simulink model "drone_sim"  (R2022a)
settings: Solver=VariableStepAuto  StartTime=0.0  StopTime=100  RelTol=1e-3
libraries: slpidlib x3
settings Model: Creator=jovanny-macbookair  LastModifiedBy=jovanny-macbookair

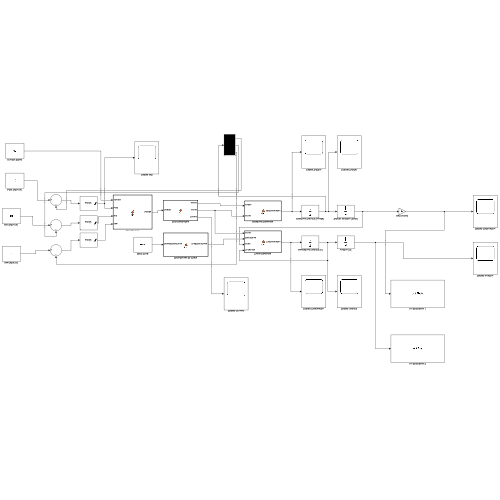
[thumbnail: Simulink's stored preview of the top-level diagram]
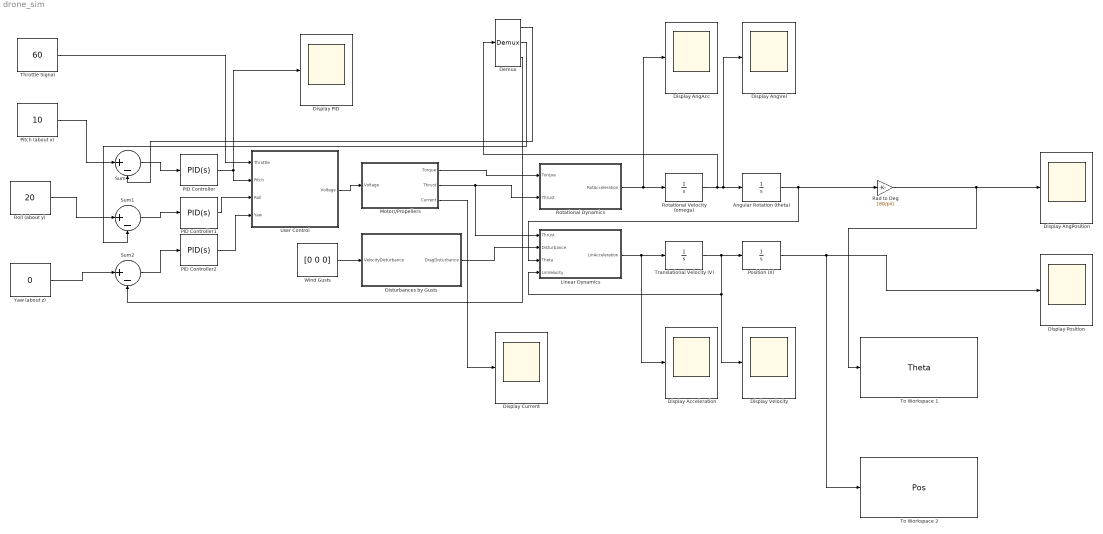
== system drone_sim ==
  Angular Rotation (theta) : Integrator
  Demux : Demux  Outputs=3
  Display Acceleration : Scope
  Display AngAcc : Scope
  Display AngPosition : Scope
  Display AngVel : Scope
  Display Current : Scope
  Display PID : Scope
  Display Position : Scope
  Display Velocity : Scope
  Disturbances by Gusts : MATLAB Function  TreatAsAtomicUnit=on
  Linear Dynamics : MATLAB Function  TreatAsAtomicUnit=on
  Motor//Propellers : MATLAB Function  TreatAsAtomicUnit=on
  PID Controller : slpidlib/PID Controller  Controller=PID  Form=Parallel  TimeDomain=Continuous-time  UseExternalTs=off  SampleTime=-1  IntegratorMethod=Forward Euler  FilterMethod=Forward Euler  ControllerParametersSource=internal  P=10  I=5  UseKiTs=off  D=0  N=100  UseFilter=on  TunerSelectOption=Transfer Function Based (PID Tuner App)  InitialConditionSource=internal  InitialConditionForIntegrator=0  InitialConditionForFilter=0  DifferentiatorICPrevScaledInput=0  ExternalReset=none  TrackingMode=off  Kt=1  LimitOutput=on  SatLimitsSource=internal  UpperSaturationLimit=100  LowerSaturationLimit=0  LinearizeAsGain=on  AntiWindupMode=clamping  Kb=1  POutMin=[]  POutMax=[]  IOutMin=[]  IOutMax=[]  DOutMin=[]  DOutMax=[]  NOutMin=[]  NOutMax=[]  SumOutMin=[]  SumOutMax=[]  SaturationOutMin=[]  SaturationOutMax=[]  PParamMin=[]  PParamMax=[]  IParamMin=[]  IParamMax=[]  DParamMin=[]  DParamMax=[]  NParamMin=[]  NParamMax=[]  KbParamMin=[]  KbParamMax=[]  KtParamMin=[]  KtParamMax=[]  KbOutMin=[]  KbOutMax=[]  KtOutMin=[]  KtOutMax=[]  IntegratorOutMin=[]  IntegratorOutMax=[]  FilterOutMin=[]  FilterOutMax=[]  SumI1OutMin=[]  SumI1OutMax=[]  SumI2OutMin=[]  SumI2OutMax=[]  SumI3OutMin=[]  SumI3OutMax=[]  SumI4OutMin=[]  SumI4OutMax=[]  SumDOutMin=[]  SumDOutMax=[]  DifferentiatorOutMin=[]  DifferentiatorOutMax=[]  FilterDiffOutCoefMin=[]  FilterDiffOutCoefMax=[]  ReciprocalOutMin=[]  ReciprocalOutMax=[]  SumDenOutMin=[]  SumDenOutMax=[]  SumNumOutMin=[]  SumNumOutMax=[]  DivideOutMin=[]  DivideOutMax=[]  UdiffTsProdOutMin=[]  UdiffTsProdOutMax=[]  NTsProdOutMin=[]  NTsProdOutMax=[]  UintegralTsProdOutMin=[]  UintegralTsProdOutMax=[]  UngainTsProdOutMin=[]  UngainTsProdOutMax=[]  IntegratorContinuousStateAttributes=''  IntegratorStateMustResolveToSignalObject=off  IntegratorRTWStateStorageClass=Auto  FilterContinuousStateAttributes=''  FilterStateMustResolveToSignalObject=off  FilterRTWStateStorageClass=Auto  ParallelPVariant=InternalParameters  IdealPVariant=Disabled  IVariant=InternalParameters  DVariant=InternalParameters  IntegratorVariant=Continuous  SatVariant=Enabled  AWVariant=ContClampingParallel  PCopyVariant=Disabled  TRVariant=Disabled  FdbkBlocksVariant=Forward  IdealPFdbkVariant=Disabled  SatFdbkVariant=Disabled  DerivativeFilterVariant=ContFilter  NVariant=InternalParameters  NCopyVariant=Disabled  FilterICVariant=InternalICsFilter  IntegratorICVariant=InternalICs  ExternalResetVariant=Disabled  TRSumVariant=Passthrough  SumFdbkVariant=Disabled  SumVariant=Sum_PID  TsampFilterVariant=InternalTs  TsampNgainVariant=Passthrough  TsampIntegralVariant=Passthrough  ExternalSaturationOutDataTypeStr=Inherit: Same as second input  aMode=0
  PID Controller1 : slpidlib/PID Controller  Controller=PID  Form=Parallel  TimeDomain=Continuous-time  UseExternalTs=off  SampleTime=-1  IntegratorMethod=Forward Euler  FilterMethod=Forward Euler  ControllerParametersSource=internal  P=10  I=5  UseKiTs=off  D=0  N=100  UseFilter=on  TunerSelectOption=Transfer Function Based (PID Tuner App)  InitialConditionSource=internal  InitialConditionForIntegrator=0  InitialConditionForFilter=0  DifferentiatorICPrevScaledInput=0  ExternalReset=none  TrackingMode=off  Kt=1  LimitOutput=on  SatLimitsSource=internal  UpperSaturationLimit=100  LowerSaturationLimit=0  LinearizeAsGain=on  AntiWindupMode=clamping  Kb=1  POutMin=[]  POutMax=[]  IOutMin=[]  IOutMax=[]  DOutMin=[]  DOutMax=[]  NOutMin=[]  NOutMax=[]  SumOutMin=[]  SumOutMax=[]  SaturationOutMin=[]  SaturationOutMax=[]  PParamMin=[]  PParamMax=[]  IParamMin=[]  IParamMax=[]  DParamMin=[]  DParamMax=[]  NParamMin=[]  NParamMax=[]  KbParamMin=[]  KbParamMax=[]  KtParamMin=[]  KtParamMax=[]  KbOutMin=[]  KbOutMax=[]  KtOutMin=[]  KtOutMax=[]  IntegratorOutMin=[]  IntegratorOutMax=[]  FilterOutMin=[]  FilterOutMax=[]  SumI1OutMin=[]  SumI1OutMax=[]  SumI2OutMin=[]  SumI2OutMax=[]  SumI3OutMin=[]  SumI3OutMax=[]  SumI4OutMin=[]  SumI4OutMax=[]  SumDOutMin=[]  SumDOutMax=[]  DifferentiatorOutMin=[]  DifferentiatorOutMax=[]  FilterDiffOutCoefMin=[]  FilterDiffOutCoefMax=[]  ReciprocalOutMin=[]  ReciprocalOutMax=[]  SumDenOutMin=[]  SumDenOutMax=[]  SumNumOutMin=[]  SumNumOutMax=[]  DivideOutMin=[]  DivideOutMax=[]  UdiffTsProdOutMin=[]  UdiffTsProdOutMax=[]  NTsProdOutMin=[]  NTsProdOutMax=[]  UintegralTsProdOutMin=[]  UintegralTsProdOutMax=[]  UngainTsProdOutMin=[]  UngainTsProdOutMax=[]  IntegratorContinuousStateAttributes=''  IntegratorStateMustResolveToSignalObject=off  IntegratorRTWStateStorageClass=Auto  FilterContinuousStateAttributes=''  FilterStateMustResolveToSignalObject=off  FilterRTWStateStorageClass=Auto  ParallelPVariant=InternalParameters  IdealPVariant=Disabled  IVariant=InternalParameters  DVariant=InternalParameters  IntegratorVariant=Continuous  SatVariant=Enabled  AWVariant=ContClampingParallel  PCopyVariant=Disabled  TRVariant=Disabled  FdbkBlocksVariant=Forward  IdealPFdbkVariant=Disabled  SatFdbkVariant=Disabled  DerivativeFilterVariant=ContFilter  NVariant=InternalParameters  NCopyVariant=Disabled  FilterICVariant=InternalICsFilter  IntegratorICVariant=InternalICs  ExternalResetVariant=Disabled  TRSumVariant=Passthrough  SumFdbkVariant=Disabled  SumVariant=Sum_PID  TsampFilterVariant=InternalTs  TsampNgainVariant=Passthrough  TsampIntegralVariant=Passthrough  ExternalSaturationOutDataTypeStr=Inherit: Same as second input  aMode=0
  PID Controller2 : slpidlib/PID Controller  Controller=PID  Form=Parallel  TimeDomain=Continuous-time  UseExternalTs=off  SampleTime=-1  IntegratorMethod=Forward Euler  FilterMethod=Forward Euler  ControllerParametersSource=internal  P=5  I=0.1  UseKiTs=off  D=0  N=100  UseFilter=on  TunerSelectOption=Transfer Function Based (PID Tuner App)  InitialConditionSource=internal  InitialConditionForIntegrator=0  InitialConditionForFilter=0  DifferentiatorICPrevScaledInput=0  ExternalReset=none  TrackingMode=off  Kt=1  LimitOutput=on  SatLimitsSource=internal  UpperSaturationLimit=100  LowerSaturationLimit=0  LinearizeAsGain=on  AntiWindupMode=clamping  Kb=1  POutMin=[]  POutMax=[]  IOutMin=[]  IOutMax=[]  DOutMin=[]  DOutMax=[]  NOutMin=[]  NOutMax=[]  SumOutMin=[]  SumOutMax=[]  SaturationOutMin=[]  SaturationOutMax=[]  PParamMin=[]  PParamMax=[]  IParamMin=[]  IParamMax=[]  DParamMin=[]  DParamMax=[]  NParamMin=[]  NParamMax=[]  KbParamMin=[]  KbParamMax=[]  KtParamMin=[]  KtParamMax=[]  KbOutMin=[]  KbOutMax=[]  KtOutMin=[]  KtOutMax=[]  IntegratorOutMin=[]  IntegratorOutMax=[]  FilterOutMin=[]  FilterOutMax=[]  SumI1OutMin=[]  SumI1OutMax=[]  SumI2OutMin=[]  SumI2OutMax=[]  SumI3OutMin=[]  SumI3OutMax=[]  SumI4OutMin=[]  SumI4OutMax=[]  SumDOutMin=[]  SumDOutMax=[]  DifferentiatorOutMin=[]  DifferentiatorOutMax=[]  FilterDiffOutCoefMin=[]  FilterDiffOutCoefMax=[]  ReciprocalOutMin=[]  ReciprocalOutMax=[]  SumDenOutMin=[]  SumDenOutMax=[]  SumNumOutMin=[]  SumNumOutMax=[]  DivideOutMin=[]  DivideOutMax=[]  UdiffTsProdOutMin=[]  UdiffTsProdOutMax=[]  NTsProdOutMin=[]  NTsProdOutMax=[]  UintegralTsProdOutMin=[]  UintegralTsProdOutMax=[]  UngainTsProdOutMin=[]  UngainTsProdOutMax=[]  IntegratorContinuousStateAttributes=''  IntegratorStateMustResolveToSignalObject=off  IntegratorRTWStateStorageClass=Auto  FilterContinuousStateAttributes=''  FilterStateMustResolveToSignalObject=off  FilterRTWStateStorageClass=Auto  ParallelPVariant=InternalParameters  IdealPVariant=Disabled  IVariant=InternalParameters  DVariant=InternalParameters  IntegratorVariant=Continuous  SatVariant=Enabled  AWVariant=ContClampingParallel  PCopyVariant=Disabled  TRVariant=Disabled  FdbkBlocksVariant=Forward  IdealPFdbkVariant=Disabled  SatFdbkVariant=Disabled  DerivativeFilterVariant=ContFilter  NVariant=InternalParameters  NCopyVariant=Disabled  FilterICVariant=InternalICsFilter  IntegratorICVariant=InternalICs  ExternalResetVariant=Disabled  TRSumVariant=Passthrough  SumFdbkVariant=Disabled  SumVariant=Sum_PID  TsampFilterVariant=InternalTs  TsampNgainVariant=Passthrough  TsampIntegralVariant=Passthrough  ExternalSaturationOutDataTypeStr=Inherit: Same as second input  aMode=0
  Pitch (about x) : Constant  Value=10
  Position (X) : Integrator
  Rad to Deg : Gain  Gain=180/pi()
  Roll (about y) : Constant  Value=20
  Rotational Dynamics : MATLAB Function  TreatAsAtomicUnit=on
  Rotational Velocity (omega) : Integrator
  Sum : Sum  Inputs=|+-
  Sum1 : Sum  Inputs=|+-
  Sum2 : Sum  Inputs=|+-
  Throttle Signal : Constant  Value=60
  To Workspace 1 : ToWorkspace  VariableName=Theta  SampleTime=0.1
      settings: Save2DSignal=2-D array (concatenate along first dimension)
  To Workspace 2 : ToWorkspace  VariableName=Pos  SampleTime=0.1
      settings: Save2DSignal=2-D array (concatenate along first dimension)
  Translational Velocity (V) : Integrator
  User Control : MATLAB Function  TreatAsAtomicUnit=on
  Wind Gusts : Constant  Value=[0 0 0]
  Yaw (about z) : Constant  Value=0
  wires:
  Motor//Propellers/1(Torque) -> Rotational Dynamics/1(Torque)
  Motor//Propellers/2(Thrust) -> Linear Dynamics/1(Thrust), Rotational Dynamics/2(Thrust)
  Rotational Dynamics/1(RotAcceleration) -> Display AngAcc/1, Rotational Velocity (omega)/1
  Rotational Velocity (omega)/1 -> Demux/1, Display AngVel/1, Angular Rotation (theta)/1
  Angular Rotation (theta)/1 -> Linear Dynamics/3(Theta), Rad to Deg/1
  Linear Dynamics/1(LinAcceleration) -> Display Acceleration/1, Translational Velocity (V)/1
  Translational Velocity (V)/1 -> Display Velocity/1, Linear Dynamics/4(LinVelocity), Position (X)/1
  Disturbances by Gusts/1(DragDisturbance) -> Linear Dynamics/2(Disturbance)
  Wind Gusts/1 -> Disturbances by Gusts/1(VelocityDisturbance)
  User Control/1(Voltage) -> Motor//Propellers/1(Voltage)
  Rad to Deg/1 -> To Workspace 1/1, Display AngPosition/1
  Motor//Propellers/3(Current) -> Display Current/1
  Position (X)/1 -> To Workspace 2/1, Display Position/1
  PID Controller/1 -> Display PID/1, User Control/2(Pitch)
  Sum/1 -> PID Controller/1
  Demux/1 -> Sum/2
  Throttle Signal/1 -> User Control/1(Throttle)
  Pitch (about x)/1 -> Sum/1
  Demux/2 -> Sum1/2
  Roll (about y)/1 -> Sum1/1
  Sum1/1 -> PID Controller1/1
  PID Controller1/1 -> User Control/3(Roll)
  Yaw (about z)/1 -> Sum2/1
  Demux/3 -> Sum2/2
  Sum2/1 -> PID Controller2/1
  PID Controller2/1 -> User Control/4(Yaw)

== matlab function drone_sim/Rotational Dynamics ==
  data: Torque input; RotAcceleration output; Thrust input
function RotAcceleration = fcn(Torque, Thrust)
Moment = [0 0 0]; 
RotAcceleration = [0 0 0]; 
MomInertia = [0.003 0.003 0.007];

% Calculate sums of Moments
Moment(1) = (Thrust(3)+Thrust(4))*0.237/2-(Thrust(1)+Thrust(2))*0.237/2; % Roll
Moment(2) = (Thrust(3)+Thrust(2))*0.237/2-(Thrust(1)+Thrust(4))*0.237/2; % Pitch
Moment(3) = Torque(4)-Torque(1)+Torque(2)-Torque(3); % Yaw

% Calculate RotAcc in all 3 directions
for i = 1:3
    RotAcceleration(i) = Moment(i)/ MomInertia(i);
end

== matlab function drone_sim/Motor////Propellers ==
  data: Voltage input; Torque output; Thrust output; Current output
function [Torque, Thrust, Current] = fcn(Voltage)
RPM = [0 0 0 0];
Torque = [0 0 0 0];
Current = [0 0 0 0];
Thrust = [0 0 0 0];

% Calculate values for all 4 propellers with respect to Voltage input
for i = 1:4
    RPM(i) = -2.6931*Voltage(i)^3 + 1400*Voltage(i);
    Ct = 2*10^-15*RPM(i)^3 - 4*10^-11*RPM(i)^2 + 3*10^-7*RPM(i) + 0.1013;
    Thrust(i) = Ct*1.225*(RPM(i)/60)^2 * (0.2^4);
    Torque(i) = 4*10^-14*RPM(i)^3 + 8*10^-12*RPM(i)^2 + 3*10^-6*RPM(i);
    Current(i) = 1400*Torque(i);
end

== matlab function drone_sim/Linear Dynamics ==
  data: Thrust input; LinAcceleration output; Disturbance input; Theta input; LinVelocity input
function LinAcceleration = fcn(Thrust, Disturbance, Theta, LinVelocity)
m = 0.743; % kg
g = 9.81; % m/s^2
A = [0.0197 0.0197 0.0512]; % m^2
rho = 1.225; % kg*m^-3
Cd = 1; % drag coefficient

LinAcceleration = [0 0 0];
Force = [0 0 0];
Fprop = [0 0 0];

% Force from propellors in 3 dimensions
Fprop(1) = sin(Theta(2))*cos(Theta(1))*(Thrust(1)+Thrust(2)+Thrust(3)+Thrust(4));
Fprop(2) = sin(Theta(1))*cos(Theta(2))*(Thrust(1)+Thrust(2)+Thrust(3)+Thrust(4));
Fprop(3) = cos(Theta(1))*cos(Theta(2))*(Thrust(1)+Thrust(2)+Thrust(3)+Thrust(4));

% Computing linear motion using X and Y vector
ThetaXY = -atan2(Fprop(1),Fprop(2)); % using "-" since our coord system is [-x, y, z]
XY2D = sqrt(Fprop(1)^2+Fprop(2)^2);

% Positive Z-direction
if Fprop(3)>=0
    Fprop(1) = XY2D*sin(ThetaXY+Theta(3));
    Fprop(2) = XY2D*cos(ThetaXY+Theta(3));
% Negative Z-direction
else
    Fprop(1) = XY2D*sin(ThetaXY-Theta(3));
    Fprop(2) = XY2D*cos(ThetaXY-Theta(3));
end

% Sum of Forces in X-direction
if LinVelocity(1) < 0
    Force(1) = Fprop(1) - Disturbance(1) + 0.5*rho*LinVelocity(1)^2*A(1)*Cd;
else
    Force(1) = Fprop(1) - Disturbance(1) - 0.5*rho*LinVelocity(1)^2*A(1)*Cd;
end

% Sum of Forces in Y-direction
if LinVelocity(2) < 0
    Force(2) = Fprop(2) - Disturbance(1) + 0.5*rho*LinVelocity(2)^2*A(2)*Cd;
else
    Force(2) = Fprop(2) - Disturbance(2) - 0.5*rho*LinVelocity(2)^2*A(2)*Cd;
end

% Sum of Forces in Z-direction
if LinVelocity(3) < 0
    Force(3) = Fprop(3) - Disturbance(3) + 0.5*rho*LinVelocity(3)^2*A(3)*Cd - m*g;
else
    Force(3) = Fprop(3) - Disturbance(3) - 0.5*rho*LinVelocity(3)^2*A(3)*Cd - m*g;
end

% Calculate LinAcc in all three directions
for i = 1:3
    LinAcceleration(i) = Force(i)/m;
end

== matlab function drone_sim/Disturbances by Gusts ==
  data: VelocityDisturbance input; DragDisturbance output
function DragDisturbance = fcn(VelocityDisturbance)
A = [0.0197 0.0197 (0.0197*2*1.33)];
DragDisturbance = [0 0 0];
rho = 1.225;
Cd = 1;

% Goal is to counter velocity of disturbance
for i = 1:3
    % if disturbance goes against drone
    if VelocityDisturbance(i) < 0
        DragDisturbance(i) = 0.5*rho*VelocityDisturbance(i)^2*A(i)*Cd;
    %if disturbance is from back of drone
    else
        DragDisturbance(i) = -0.5*rho*VelocityDisturbance(i)^2*A(i)*Cd;
    end
end

== matlab function drone_sim/User Control ==
  data: Throttle input; Voltage output; Pitch input; Roll input; Yaw input
function Voltage = fcn(Throttle, Pitch, Roll, Yaw)
Correct = 0;
% function fits input into our throttle system
% drone throttle system: 10 - 100%, where 10 is 0% for us
% divide by 2 since we have two motors
if (Pitch/2+Roll/2+Yaw/2)>(100-Throttle) 
    Correct = ((Pitch/2+Roll/2+Yaw/2)-(100-Throttle));
end
if (Pitch/2+Roll/2+Yaw/2)>(Throttle)
    if Correct<((Pitch/2+Roll/2+Yaw/2)-(Throttle))
        Correct = ((Pitch/2+Roll/2+Yaw/2)-(Throttle));
    end
end

% correct the inputs using system's algorithm
% subtract excess input amongst all three motions
% multiply by 2 to account for both motors
if Correct ~= 0
Pitch = Pitch-Correct/3*2;
Roll = Roll-Correct/3*2;
Yaw = Yaw-Correct/3*2;
end

Voltage = [(Throttle-Pitch/2-Roll/2-Yaw/2)*11.4/100
    (Throttle-Pitch/2+Roll/2+Yaw/2)*11.4/100
    (Throttle+Pitch/2+Roll/2-Yaw/2)*11.4/100
    (Throttle+Pitch/2-Roll/2+Yaw/2)*11.4/100];
